simulink model "example_Storage_type1conf"  (R2016b)
settings: Solver=ode45  StartTime=0.0  StopTime=3*3600-2  MaxStep=300  RelTol=1e-3  EnableMultiTasking=on
undefined symbols (not defined in the file): path_carnot
libraries: carnot x10, simulink x2
settings Model: Creator=drhf  LastModifiedBy=drhf
settings DataIOCC: LimitDataPoints=on  SaveFormat=Array
settings OptimizationCC: ExpressionDepthLimit=2147483647  LifeSpan=inf
settings DebuggingCC: UnderspecifiedInitializationDetection=Classic  MergeDetectMultiDrivingBlocksExec=none  SolverPrmCheckMsg=warning  StateNameClashWarn=warning  SFUnexpectedBacktrackingDiag=warning  SFNoUnconditionalDefaultTransitionDiag=warning  SFExecutionAtInitializationDiag=none
settings HardwareCC: ProdBitPerPointer=32  ProdBitPerSizeT=32  ProdBitPerPtrDiffT=32  ProdLargestAtomicFloat=None  ProdIntDivRoundTo=Undefined  ProdEndianess=Unspecified  ProdWordSize=32  ProdHWDeviceType=32-bit Generic
settings ModelReferenceCC: PropagateSignalLabelsOutOfModel=off
settings GRTTargetCC: TargetLangStandard=C89/C90 (ANSI)  GeneratePreprocessorConditionals=Disable all  CombineOutputUpdateFcns=off  GRTInterface=on
settings ConfigComp: CovMetricSettings=dw  CovHtmlReporting=on  CovSaveCumulativeToWorkspaceVar=on  CovSaveSingleToWorkspaceVar=on  CovExternalEMLEnable=off

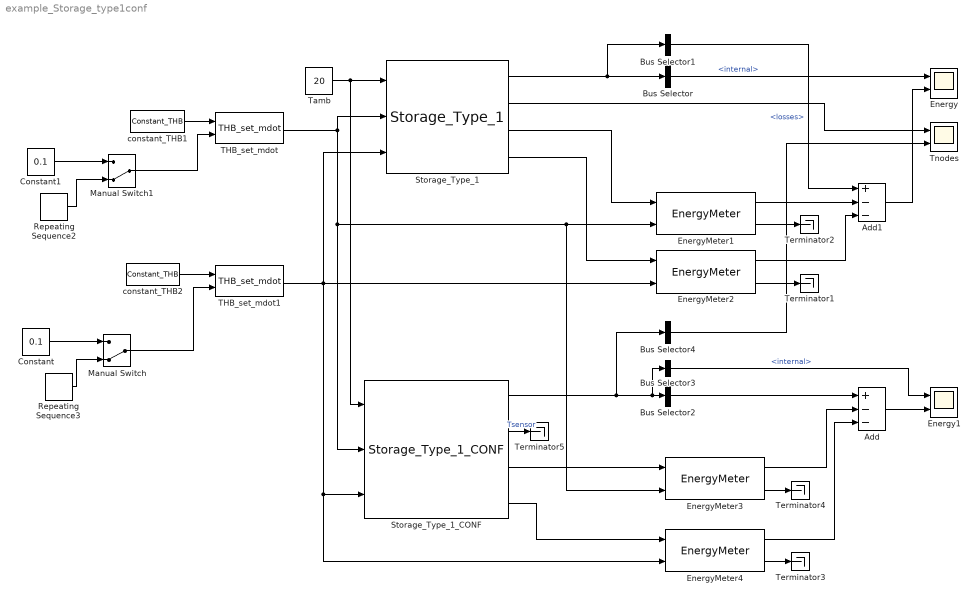
== system example_Storage_type1conf ==
  Add : Sum  Inputs=+--
  Add1 : Sum  Inputs=+--
  Bus Selector : BusSelector  OutputSignals=energy.internal
  Bus Selector1 : BusSelector  OutputSignals=energy.losses
  Bus Selector2 : BusSelector  OutputSignals=energy.losses  OutputAsBus=on
  Bus Selector3 : BusSelector  OutputSignals=energy.internal
  Bus Selector4 : BusSelector  OutputSignals=Tnodes  OutputAsBus=on
  Constant : Constant  Value=0.1
  Constant1 : Constant  Value=0.1
  Energy : Scope  NumInputPorts=2
  Energy1 : Scope  NumInputPorts=2
  EnergyMeter{1..4} (4 alike) : carnot/Control/EnergyMeter
  Manual Switch : ManualSwitch  CurrentSetting=0
  Manual Switch1 : ManualSwitch  CurrentSetting=0
  Repeating Sequence2 : simulink/Sources/Repeating Sequence  rep_seq_t=[ 0 3600 3600+eps(3600) 7200 7200+eps(7200) 10440 10440+eps(10440) 11160]  rep_seq_y=[ 0.12 0.12 0.15+0*eps(3600) 0.15 0.1+0*eps(7200) 0.1 0+0*eps(10440) 0]
  Repeating Sequence3 : simulink/Sources/Repeating Sequence  rep_seq_t=[ 0 3600 3600+eps(3600) 7200 7200+eps(7200) 10800]  rep_seq_y=[ 0.12 0.12 0.1+0*eps(3600) 0.1 0.15+0*eps(7200) 0.15]
  Storage_Type_1 : carnot/Storage/Thermal/Storage_Type_1  uloss=1  ubot=1  utop=1  cond=1  volume=0.3  dia=0.5  pos=standing cylinder  h_in_chg=1  h_out_chg=0  pipe1dia=0.03  h_in=0  h_out=1  pipe2dia=0.03  t0=[10:5:55]  nodes=10  mpoints=10
  Storage_Type_1_CONF : carnot/Storage/Thermal/Storage_Type_1_CONF  t0=[10:5:55]  tini=[10 15 20 25 30 35 40 45 50 55]  hgt=1.7684  mpts=[1 2 3 4 5 6 7 8 9 10]  PathName=fullfile(path_carnot('libsl'),'Storage','Thermal','Storage_Type_1_CONF','parameter_set')  FileName='StorageType1_500_L.mat'  userPath=off  userParam=off  uwall=1  ubot=1  utop=1  axcond=1  volume=0.5  dia=0.6  standing=standing cylinder  nodes=10  mpoints=10  Tsensor=0.5  pipe3inlet=1  pipe3outlet=0  pipe3dia=0.03  pipe2inlet=0  pipe2outlet=1  pipe2dia=0.03
  THB_set_mdot : carnot/Source/Simple/THB_set_mdot
  THB_set_mdot1 : carnot/Source/Simple/THB_set_mdot
  Tamb : Constant  Value=20
  Terminator{1..5} (5 alike) : Terminator
  Tnodes : Scope  NumInputPorts=2
  constant_THB1 : carnot/Source/Simple/Constant_THB  t=55  mdot=0*100/3600  p=1e5  mID=Full Pressure Drop with Static Height  fluid=Water  mix=0  mix2=0  mix3=0  dia=0.02  hgt=0
  constant_THB2 : carnot/Source/Simple/Constant_THB  t=10  mdot=100/3600  p=1e5  mID=Full Pressure Drop with Static Height  fluid=Water  mix=0  mix2=0  mix3=0  dia=0.02  hgt=0
  wires:
  Bus Selector/1 -> Energy/1  "<internal>"
  Tamb/1 -> Storage_Type_1_CONF/1, Storage_Type_1/1
  THB_set_mdot/1 -> Storage_Type_1_CONF/2, EnergyMeter3/2, EnergyMeter1/2, Storage_Type_1/2
  THB_set_mdot1/1 -> EnergyMeter4/2, Storage_Type_1_CONF/3, EnergyMeter2/2, Storage_Type_1/3
  Storage_Type_1/1 -> Bus Selector1/1, Bus Selector/1
  Storage_Type_1/2 -> Tnodes/1
  Storage_Type_1/3 -> EnergyMeter1/1
  Storage_Type_1/4 -> EnergyMeter2/1
  EnergyMeter2/2 -> Terminator1/1
  constant_THB1/1 -> THB_set_mdot/1
  constant_THB2/1 -> THB_set_mdot1/1
  Manual Switch1/1 -> THB_set_mdot/2
  Manual Switch/1 -> THB_set_mdot1/2
  Constant/1 -> Manual Switch/1
  Repeating Sequence3/1 -> Manual Switch/2
  Constant1/1 -> Manual Switch1/1
  Repeating Sequence2/1 -> Manual Switch1/2
  EnergyMeter1/2 -> Terminator2/1
  EnergyMeter2/1 -> Add1/3
  EnergyMeter1/1 -> Add1/2
  Storage_Type_1_CONF/3 -> EnergyMeter3/1
  EnergyMeter3/1 -> Add/2
  EnergyMeter4/1 -> Add/3
  Storage_Type_1_CONF/1 -> Bus Selector3/1, Bus Selector2/1, Bus Selector4/1
  Storage_Type_1_CONF/4 -> EnergyMeter4/1
  EnergyMeter4/2 -> Terminator3/1
  EnergyMeter3/2 -> Terminator4/1
  Bus Selector4/1 -> Tnodes/2
  Storage_Type_1_CONF/2 -> Terminator5/1  "Tsensor"
  Bus Selector1/1 -> Add1/1  "<losses>"
  Add1/1 -> Energy/2
  Bus Selector2/1 -> Add/1
  Add/1 -> Energy1/2
  Bus Selector3/1 -> Energy1/1  "<internal>"
